simulink model "PubIfDecisionLM_MDL"  (R2020b)
settings: configuration reference "DspaceConfig" (kept outside this file)
PostLoadFcn:
  | if any(exist('dsrtsu_mdlpostloadfcn', 'file') ~= 0), dsrtsu_mdlpostloadfcn('Execute', bdroot); end
InitFcn:
  | , if any(exist('dsmpb_private', 'file') ~= 0), dsmpb_private('dsmpb_mdlclblib', 'Init', bdroot); end,
undefined symbols (not defined in the file or in its folder): OFM_OBJ_FUSIONTYPE_E, OFM_OBJ_MOVINGSTATE_E, OFM_OBJ_ORIENTATION_E, OFM_OBJ_TYPE_E, P_LM_Cyc, P_LM_EMLHistKapRcdBufSize, P_LM_EMLHistTrajBaseDis, P_LM_EMLHistTrajPNum, P_LM_EMLKapCorrMaxThre, P_LM_EMLMinKapThre, P_LM_EMLPathDisDiffThre, P_LM_EMLQuaFiltPar, P_LM_EMLTurnActKapThre, P_LM_EMLValidQuaThre, P_LM_FntPath1Disgap, P_LM_FntPath1MinDis, P_LM_FntPath1Timegap, P_LM_FntPath2Disgap, P_LM_FntPath2MinDis, P_LM_FntPath2Timegap, P_LM_FntPath3Disgap, P_LM_FntPath3MinDis, P_LM_FntPath3Timegap, P_LM_FusBLParFiltP, P_LM_FusEVDifC2Thre, P_LM_FusEVOPath1AllVSLDisThre, P_LM_FusEVOPath1AllVSLLostNumThre, P_LM_FusEVOPath1AllVSLQuaThre, P_LM_FusEVOPath1OTLFacNLC, P_LM_FusOTLQuaThre, P_LM_FusOTLSW, P_LM_FusParC0Index, P_LM_FusParC1Index, P_LM_FusParC2Index, P_LM_FusParC3Index, P_LM_FusVSLQuaThre, P_LM_FusVSLSW, P_LM_FusVSLValidSteerWheerAngThre, P_LM_FusVSLValidVxvThre, P_LM_LaneWidth, P_LM_OTLBufTPInfoEvaFactor, P_LM_OTLObjNum, P_LM_OTLObjSelectAgeThre, P_LM_OTLObjSelectDxAssessVx, P_LM_OTLObjSelectDxThre, P_LM_OTLObjSelectVxThre, P_LM_OTLObjSelectVyAssessDx, P_LM_OTLObjSelectVyThre, P_LM_OTLTrajPntBaseDis, P_LM_OTLTrajStdThre, P_LM_VSLAvailLineNum, P_LM_VSLBLSDiffThre, P_LM_VSLBLSDisRatio, P_LM_VSLFusBLParFiltP_C1, P_LM_VSLFusBLParFiltP_C2, P_LM_VSLFusBLParFiltP_C3, P_LM_VSLFusBLParFiltP_Quality, P_LM_VSLHistTrajBaseDis, P_LM_VSLHistTrajPNum, P_LM_VSLLCC0diff ... (+18)
libraries: simulink x145, LM_LIB x43
(part 9 of 24)

== system PubIfDecisionLM_MDL/Subsystem2/LM_OTL/LM_OTL_MovObjTrajRecord3/LM_OTL_BufRcdObjLostJudge/LM_OTL_RigLaRcdObjLostJudge ==
  Object_ID : Inport  BusOutputAsStruct=on
  LM_OTLRcdObjIDVectK1 : Inport  Port=2
  LM_OTLInterestObjIndexVect : Inport  Port=3
  Bus Selector : BusSelector  OutputSignals=LM_OTLCurRigLaObj1Index,LM_OTLCurRigLaObj2Index
  Bus Selector1 : BusSelector  OutputSignals=LM_OTLBufObjIDInfo.LM_OTLBufR1ObjID,LM_OTLBufObjIDInfo.LM_OTLBufR2ObjID
  Compare To Zero : simulink/Logic and Bit Operations/Compare To Zero  relop===  OutDataTypeStr=boolean
  Compare To Zero1 : simulink/Logic and Bit Operations/Compare To Zero  relop===  OutDataTypeStr=boolean
  Compare To Zero2 : simulink/Logic and Bit Operations/Compare To Zero  relop=~=  OutDataTypeStr=boolean
  Compare To Zero3 : simulink/Logic and Bit Operations/Compare To Zero  relop===  OutDataTypeStr=boolean
  Constant : Constant  OutDataTypeStr=uint8
  Constant1 : Constant  OutDataTypeStr=uint8
  Constant2 : Constant  Value=0  OutDataTypeStr=boolean
  Constant3 : Constant  Value=0  OutDataTypeStr=boolean
  Constant4 : Constant  Value=0  OutDataTypeStr=uint8
  Index Vector2 : MultiPortSwitch  Inputs=1
  Index Vector3 : MultiPortSwitch  Inputs=1
  Logical Operator : Logic  Operator=OR  AllPortsSameDT=off  OutDataTypeStr=boolean
  Logical Operator1 : Logic  Operator=OR  AllPortsSameDT=off  OutDataTypeStr=boolean
  Logical Operator2 : Logic  Operator=NOT  AllPortsSameDT=off  OutDataTypeStr=boolean
  Logical Operator3 : Logic  Operator=NOT  AllPortsSameDT=off  OutDataTypeStr=boolean
  Relational Operator{,1..3} (4 alike) : RelationalOperator  Operator===  OutDataTypeStr=boolean  RndMeth=Simplest
  Switch{,1..5} (6 alike) : Switch  Criteria=u2 ~= 0
  LM_OTLBufRig1ObjLostFlg : Outport
  LM_OTLBufRig2ObjLostFlg : Outport  Port=2
  wires:
  Constant3/1 -> Switch5/1
  Switch5/1 -> LM_OTLBufRig1ObjLostFlg/1  "LM_OTLBufRig1ObjLostFlg"
  Compare To Zero3/1 -> Switch5/2
  Constant2/1 -> Switch4/3
  Compare To Zero2/1 -> Switch4/2
  Switch4/1 -> LM_OTLBufRig2ObjLostFlg/1  "LM_OTLBufRig2ObjLostFlg"
  LM_OTLRcdObjIDVectK1/1 -> Bus Selector1/1
  Constant1/1 -> Switch2/1
  Index Vector3/1 -> Switch3/3
  Compare To Zero1/1 -> Switch2/2, Switch3/2
  Bus Selector/2 -> Compare To Zero1/1, Switch2/3  "<LM_OTLCurRigLaObj2Index>"
  Index Vector2/1 -> Switch1/3
  Constant4/1 -> Switch1/1, Switch3/1
  LM_OTLInterestObjIndexVect/1 -> Bus Selector/1
  Compare To Zero/1 -> Switch1/2, Switch/2
  Switch/1 -> Index Vector2/1
  Switch1/1 -> Relational Operator/1, Relational Operator1/1  "LM_Rig1ObjID"
  Logical Operator3/1 -> Switch5/3
  Object_ID/1 -> Index Vector2/2, Index Vector3/2
  Constant/1 -> Switch/1
  Bus Selector1/1 -> Relational Operator2/2, Relational Operator/2, Compare To Zero3/1  "<LM_OTLBufR1ObjID>"
  Switch3/1 -> Relational Operator2/1, Relational Operator3/1  "LM_Rig2ObjID"
  Bus Selector/1 -> Compare To Zero/1, Switch/3  "<LM_OTLCurRigLaObj1Index>"
  Bus Selector1/2 -> Compare To Zero2/1, Relational Operator3/2, Relational Operator1/2  "<LM_OTLBufR2ObjID>"
  Switch2/1 -> Index Vector3/1
  Relational Operator/1 -> Logical Operator/1
  Logical Operator2/1 -> Switch4/1
  Relational Operator2/1 -> Logical Operator/2
  Relational Operator1/1 -> Logical Operator1/1
  Relational Operator3/1 -> Logical Operator1/2
  Logical Operator1/1 -> Logical Operator2/1
  Logical Operator/1 -> Logical Operator3/1

== system PubIfDecisionLM_MDL/Subsystem2/LM_OTL/LM_OTL_MovObjTrajRecord3/LM_OTL_BufTPCC/Subsystem ==
  VehStandstill : Inport
  LM_OTLOffsetX : Inport  Port=2
  LM_OTLOffsetY : Inport  Port=3
  LM_OTLOffsetAng : Inport  Port=4
  LM_OTLBufL1DxVectK1 : Inport  Port=5
  LM_OTLBufL1DyVectK1 : Inport  Port=6
  LM_OTLBufL2DxVectK1 : Inport  Port=7
  LM_OTLBufL2DyVectK1 : Inport  Port=8
  LM_OTLBufE1DxVectK1 : Inport  Port=9
  LM_OTLBufE1DyVectK1 : Inport  Port=10
  LM_OTLBufE2DxVectK1 : Inport  Port=11
  LM_OTLBufE2DyVectK1 : Inport  Port=12
  LM_OTLBufR1DxVectK1 : Inport  Port=13
  LM_OTLBufR1DyVectK1 : Inport  Port=14
  LM_OTLBufR2DxVectK1 : Inport  Port=15
  LM_OTLBufR2DyVectK1 : Inport  Port=16
  LM_OTLHostBufCoordinateConvert : Subsystem
  LM_OTLLeBufCoordinateConvert : Subsystem
  LM_OTLRiBufCoordinateConvert : Subsystem
  LM_OTLBufL1DxVectK1Adju : Outport
  LM_OTLBufL1DyVectK1Adju : Outport  Port=2
  LM_OTLBufL2DxVectK1Adju : Outport  Port=3
  LM_OTLBufL2DyVectK1Adju : Outport  Port=4
  LM_OTLBufE1DxVectK1Adju : Outport  Port=5
  LM_OTLBufE1DyVectK1Adju : Outport  Port=6
  LM_OTLBufE2DxVectK1Adju : Outport  Port=7
  LM_OTLBufE2DyVectK1Adju : Outport  Port=8
  LM_OTLBufR1DxVectK1Adju : Outport  Port=9
  LM_OTLBufR1DyVectK1Adju : Outport  Port=10
  LM_OTLBufR2DxVectK1Adju : Outport  Port=11
  LM_OTLBufR2DyVectK1Adju : Outport  Port=12
  wires:
  LM_OTLOffsetAng/1 -> LM_OTLLeBufCoordinateConvert/4(LM_OTLOffsetAng), LM_OTLHostBufCoordinateConvert/4(LM_OTLOffsetAng), LM_OTLRiBufCoordinateConvert/4(LM_OTLOffsetAng)
  LM_OTLBufL2DxVectK1/1 -> LM_OTLLeBufCoordinateConvert/7(LM_OTLBufL2DxVectK1)
  LM_OTLOffsetX/1 -> LM_OTLLeBufCoordinateConvert/2(LM_OTLOffsetX), LM_OTLHostBufCoordinateConvert/2(LM_OTLOffsetX), LM_OTLRiBufCoordinateConvert/2(LM_OTLOffsetX)
  LM_OTLBufE2DxVectK1/1 -> LM_OTLHostBufCoordinateConvert/7(LM_OTLBufE2DxVectK1)
  LM_OTLHostBufCoordinateConvert/3(LM_OTLBufE2DxVectK1Adju) -> LM_OTLBufE2DxVectK1Adju/1
  LM_OTLLeBufCoordinateConvert/1(LM_OTLBufL1DxVectK1Adju) -> LM_OTLBufL1DxVectK1Adju/1
  VehStandstill/1 -> LM_OTLRiBufCoordinateConvert/1(VehStandstill), LM_OTLHostBufCoordinateConvert/1(VehStandstill), LM_OTLLeBufCoordinateConvert/1(VehStandstill)
  LM_OTLBufR2DyVectK1/1 -> LM_OTLRiBufCoordinateConvert/8(LM_OTLBufR2DyVectK1)
  LM_OTLLeBufCoordinateConvert/4(LM_OTLBufL2DyVectK1Adju) -> LM_OTLBufL2DyVectK1Adju/1
  LM_OTLBufE1DxVectK1/1 -> LM_OTLHostBufCoordinateConvert/5(LM_OTLBufE1DxVectK1)
  LM_OTLBufR2DxVectK1/1 -> LM_OTLRiBufCoordinateConvert/7(LM_OTLBufR2DxVectK1)
  LM_OTLBufE1DyVectK1/1 -> LM_OTLHostBufCoordinateConvert/6(LM_OTLBufE1DyVectK1)
  LM_OTLRiBufCoordinateConvert/3(LM_OTLBufR2DxVectK1Adju) -> LM_OTLBufR2DxVectK1Adju/1
  LM_OTLHostBufCoordinateConvert/4(LM_OTLBufE2DyVectK1Adju) -> LM_OTLBufE2DyVectK1Adju/1
  LM_OTLRiBufCoordinateConvert/4(LM_OTLBufR2DyVectK1Adju) -> LM_OTLBufR2DyVectK1Adju/1
  LM_OTLBufL1DyVectK1/1 -> LM_OTLLeBufCoordinateConvert/6(LM_OTLBufL1DyVectK1)
  LM_OTLBufR1DxVectK1/1 -> LM_OTLRiBufCoordinateConvert/5(LM_OTLBufR1DxVectK1)
  LM_OTLOffsetY/1 -> LM_OTLHostBufCoordinateConvert/3(LM_OTLOffsetY), LM_OTLRiBufCoordinateConvert/3(LM_OTLOffsetY), LM_OTLLeBufCoordinateConvert/3(LM_OTLOffsetY)
  LM_OTLBufR1DyVectK1/1 -> LM_OTLRiBufCoordinateConvert/6(LM_OTLBufR1DyVectK1)
  LM_OTLBufL2DyVectK1/1 -> LM_OTLLeBufCoordinateConvert/8(LM_OTLBufL2DyVectK1)
  LM_OTLHostBufCoordinateConvert/1(LM_OTLBufE1DxVectK1Adju) -> LM_OTLBufE1DxVectK1Adju/1
  LM_OTLRiBufCoordinateConvert/1(LM_OTLBufR1DxVectK1Adju) -> LM_OTLBufR1DxVectK1Adju/1
  LM_OTLLeBufCoordinateConvert/3(LM_OTLBufL2DxVectK1Adju) -> LM_OTLBufL2DxVectK1Adju/1
  LM_OTLRiBufCoordinateConvert/2(LM_OTLBufR1DyVectK1Adju) -> LM_OTLBufR1DyVectK1Adju/1
  LM_OTLHostBufCoordinateConvert/2(LM_OTLBufE1DyVectK1Adju) -> LM_OTLBufE1DyVectK1Adju/1
  LM_OTLLeBufCoordinateConvert/2(LM_OTLBufL1DyVectK1Adju) -> LM_OTLBufL1DyVectK1Adju/1
  LM_OTLBufE2DyVectK1/1 -> LM_OTLHostBufCoordinateConvert/8(LM_OTLBufE2DyVectK1)
  LM_OTLBufL1DxVectK1/1 -> LM_OTLLeBufCoordinateConvert/5(LM_OTLBufL1DxVectK1)

== system PubIfDecisionLM_MDL/Subsystem2/LM_OTL/LM_OTL_MovObjTrajRecord3/LM_OTL_MovObjSelc/LM_OTL_MovObjInterestedSelc ==
  LM_OTL_MovObjValid : Inport
  P_LM_ObjNum : Inport  Port=2
  Object_DX : Inport  Port=3
  Object_DY : Inport  Port=4
  For Iterator : ForIterator  IterationSource=external
  LM_OTL_ObjSelcIndexCalc : Subsystem
  LM_OTL_ObjSelcIndexCheck : Subsystem
  LM_OTL_ObjSelcInfoCalc : Subsystem
  LM_OTLLeObj1Index : Outport
  LM_OTLLeObj2Index : Outport  Port=2
  LM_OTLHostObj1Index : Outport  Port=3
  LM_OTLHostObj2Index : Outport  Port=4
  LM_OTLRigObj1Index : Outport  Port=5
  LM_OTLRigObj2Index : Outport  Port=6
  wires:
  LM_OTL_ObjSelcIndexCheck/3(LM_OTLHostObj1Index) -> LM_OTLHostObj1Index/1
  [ObjDy] -> LM_OTL_ObjSelcIndexCheck/8(Object_DX)
  [ObjValid] -> LM_OTL_ObjSelcIndexCheck/7(LM_OTL_MovObjValid)
  LM_OTL_ObjSelcIndexCalc/6(RigObj2CheckInfo) -> LM_OTL_ObjSelcIndexCheck/6(RigObj2CheckInfo)
  LM_OTL_ObjSelcIndexCalc/5(RigObj1CheckInfo) -> LM_OTL_ObjSelcIndexCheck/5(RigObj1CheckInfo)
  LM_OTL_ObjSelcIndexCalc/4(HostObj2CheckInfo) -> LM_OTL_ObjSelcIndexCheck/4(HostObj2CheckInfo)
  LM_OTL_ObjSelcIndexCalc/3(HostObj1CheckInfo) -> LM_OTL_ObjSelcIndexCheck/3(HostObj1CheckInfo)
  LM_OTL_ObjSelcIndexCalc/2(LeObj2CheckInfo) -> LM_OTL_ObjSelcIndexCheck/2(LeObj2CheckInfo)
  LM_OTL_ObjSelcIndexCalc/1(LeObj1CheckInfo) -> LM_OTL_ObjSelcIndexCheck/1(LeObj1CheckInfo)
  LM_OTL_ObjSelcIndexCheck/6(LM_OTLRigObj2Index) -> LM_OTLRigObj2Index/1
  LM_OTL_ObjSelcIndexCheck/5(LM_OTLRigObj1Index) -> LM_OTLRigObj1Index/1
  LM_OTL_ObjSelcIndexCheck/4(LM_OTLHostObj2Index) -> LM_OTLHostObj2Index/1
  LM_OTL_ObjSelcIndexCheck/2(LM_OTLLeObj2Index) -> LM_OTLLeObj2Index/1
  LM_OTL_ObjSelcIndexCheck/1(LM_OTLLeObj1Index) -> LM_OTLLeObj1Index/1
  LM_OTL_ObjSelcInfoCalc/2(ObjSelcDyInfo) -> LM_OTL_ObjSelcIndexCalc/2(ObjSelcDyInfo)
  LM_OTL_ObjSelcInfoCalc/1(ObjSelcDxInfo) -> LM_OTL_ObjSelcIndexCalc/1(ObjSelcDxInfo)
  Object_DY/1 -> LM_OTL_ObjSelcInfoCalc/3(Object_DY), [ObjDy]
  Object_DX/1 -> LM_OTL_ObjSelcInfoCalc/2(Object_DX)
  LM_OTL_MovObjValid/1 -> LM_OTL_ObjSelcInfoCalc/1(ILM_OTL_MovObjValid), [ObjValid]
  For Iterator/1 -> LM_OTL_ObjSelcInfoCalc/4(C_LM_ObjNum), LM_OTL_ObjSelcIndexCalc/3(C_LM_ObjNum)
  P_LM_ObjNum/1 -> For Iterator/1

== system PubIfDecisionLM_MDL/Subsystem2/LM_OTL/LM_OTL_MovObjTrajRecord3/LM_OTL_MovObjSelc/Subsystem3 ==
  vxvRefMs : Inport
  <Object_ID> : Inport  Port=2  Partition=on  PartitionDimension=1  PartitionWidth=1  PartitionOffset=0
  <Object_Type> : Inport  Port=3  Partition=on  PartitionDimension=1  PartitionWidth=1  PartitionOffset=0
  <Object_MovingState> : Inport  Port=4  Partition=on  PartitionDimension=1  PartitionWidth=1  PartitionOffset=0
  <Object_VX> : Inport  Port=5  Partition=on  PartitionDimension=1  PartitionWidth=1  PartitionOffset=0
  <Object_Orientation> : Inport  Port=6  Partition=on  PartitionDimension=1  PartitionWidth=1  PartitionOffset=0
  <Object_Fus_Type> : Inport  Port=7  Partition=on  PartitionDimension=1  PartitionWidth=1  PartitionOffset=0
  <Object_ExistProb> : Inport  Port=8  Partition=on  PartitionDimension=1  PartitionWidth=1  PartitionOffset=0
  <Object_VY> : Inport  Port=9  Partition=on  PartitionDimension=1  PartitionWidth=1  PartitionOffset=0
  <Object_DX> : Inport  Port=10  Partition=on  PartitionDimension=1  PartitionWidth=1  PartitionOffset=0
  <Object_Age> : Inport  Port=11  Partition=on  PartitionDimension=1  PartitionWidth=1  PartitionOffset=0
  For Each : ForEach  DisableCoverage=on
  ILM_OTL_MovObjSelectDeFault : Subsystem  TreatAsAtomicUnit=on
  If : If  IfExpression=u1
  LM_OTL_MovObjSelect : Subsystem  TreatAsAtomicUnit=on
  Merge : Merge
  ObjIsInvalidCalc : Subsystem
  LM_OTL_MovObjValid : Outport  ConcatenationDimension=1
  wires:
  <Object_Type>/1 -> LM_OTL_MovObjSelect/2(Object_Type)
  <Object_VY>/1 -> LM_OTL_MovObjSelect/8(Object_VY)
  <Object_VX>/1 -> LM_OTL_MovObjSelect/4(Object_VX)
  <Object_DX>/1 -> LM_OTL_MovObjSelect/9(Object_DX)
  <Object_ID>/1 -> ObjIsInvalidCalc/1(ObjectID)
  <Object_MovingState>/1 -> LM_OTL_MovObjSelect/3(Object_MovingState)
  <Object_Fus_Type>/1 -> LM_OTL_MovObjSelect/6(Object_Fus_Type)
  ILM_OTL_MovObjSelectDeFault/1(LM_OTL_MovObjValid) -> Merge/1
  If/1 -> ILM_OTL_MovObjSelectDeFault/Action
  <Object_Age>/1 -> LM_OTL_MovObjSelect/10(Object_Age)
  If/2 -> LM_OTL_MovObjSelect/Action
  LM_OTL_MovObjSelect/1(LM_OTL_MovObjValid) -> Merge/2
  ObjIsInvalidCalc/1(ObjIsInvalid) -> If/1
  <Object_Orientation>/1 -> LM_OTL_MovObjSelect/5(Object_Orientation)
  <Object_ExistProb>/1 -> LM_OTL_MovObjSelect/7(Object_ExistProb)
  Merge/1 -> LM_OTL_MovObjValid/1
  vxvRefMs/1 -> LM_OTL_MovObjSelect/1(vxvRefMs)

== system PubIfDecisionLM_MDL/Subsystem2/LM_OTL/LM_OTL_MovObjTrajRecord3/LM_OTL_ObjAlreadyRcdedJudge/LM_OTL_CurObjIDCalc ==
  Object_ID : Inport  BusOutputAsStruct=on
  LM_OTLCurLeLaObj1Index : Inport  Port=2
  LM_OTLCurLeLaObj2Index : Inport  Port=3
  LM_OTLCurEgoLaObj1Index : Inport  Port=4
  LM_OTLCurEgoLaObj2Index : Inport  Port=5
  LM_OTLCurRigLaObj1Index : Inport  Port=6
  LM_OTLCurRigLaObj2Index : Inport  Port=7
  LM_OTL_CurEgoLaObjID : Subsystem
  LM_OTL_CurLeLaObjID : Subsystem
  LM_OTL_RigEgoLaObjID : Subsystem
  LM_OTLCurLeLaObj1ID : Outport
  LM_OTLCurLeLaObj2ID : Outport  Port=2
  LM_OTLCurEgoLaObj1ID : Outport  Port=3
  LM_OTLCurEgoLaObj2ID : Outport  Port=4
  LM_OTLCurRigLaObj1ID : Outport  Port=5
  LM_OTLCurRigLaObj2ID : Outport  Port=6
  wires:
  LM_OTL_CurLeLaObjID/2(LM_OTLCurLeLaObj2ID) -> LM_OTLCurLeLaObj2ID/1
  LM_OTL_CurEgoLaObjID/2(LM_OTLCurEgoLaObj2ID) -> LM_OTLCurEgoLaObj2ID/1
  LM_OTL_CurEgoLaObjID/1(LM_OTLCurEgoLaObj1ID) -> LM_OTLCurEgoLaObj1ID/1
  LM_OTL_RigEgoLaObjID/1(LM_OTLCurRigLaObj1ID) -> LM_OTLCurRigLaObj1ID/1
  LM_OTL_RigEgoLaObjID/2(LM_OTLCurRigLaObj2ID) -> LM_OTLCurRigLaObj2ID/1
  LM_OTL_CurLeLaObjID/1(LM_OTLCurLeLaObj1ID) -> LM_OTLCurLeLaObj1ID/1
  Object_ID/1 -> LM_OTL_RigEgoLaObjID/1(Object_ID), LM_OTL_CurEgoLaObjID/1(Object_ID), LM_OTL_CurLeLaObjID/1(Object_ID)
  LM_OTLCurLeLaObj2Index/1 -> LM_OTL_CurLeLaObjID/3(LM_OTLCurLeLaObj2Index)
  LM_OTLCurLeLaObj1Index/1 -> LM_OTL_CurLeLaObjID/2(LM_OTLCurLeLaObj1Index)
  LM_OTLCurEgoLaObj1Index/1 -> LM_OTL_CurEgoLaObjID/2(LM_OTLCurEgoLaObj1Index)
  LM_OTLCurEgoLaObj2Index/1 -> LM_OTL_CurEgoLaObjID/3(LM_OTLCurEgoLaObj2Index)
  LM_OTLCurRigLaObj1Index/1 -> LM_OTL_RigEgoLaObjID/2(LM_OTLCurRigLaObj1Index)
  LM_OTLCurRigLaObj2Index/1 -> LM_OTL_RigEgoLaObjID/3(LM_OTLCurRigLaObj2Index)

== system PubIfDecisionLM_MDL/Subsystem2/LM_OTL/LM_OTL_MovObjTrajRecord3/LM_OTL_ObjAlreadyRcdedJudge/LM_OTL_EglLaneRcdJudge ==
  LM_OTLCurEgoLa1ObjID : Inport
  LM_OTLCurEgoLa2ObjID : Inport  Port=2
  LM_OTLBufE1ObjIDK1 : Inport  Port=3
  LM_OTLBufE2ObjIDK1 : Inport  Port=4
  Compare To Zero : simulink/Logic and Bit Operations/Compare To Zero  relop===  OutDataTypeStr=boolean
  Compare To Zero1 : simulink/Logic and Bit Operations/Compare To Zero  relop===  OutDataTypeStr=boolean
  Constant{1..2,6,9} (4 alike) : Constant  Value=0  OutDataTypeStr=uint8
  Constant4 : Constant  OutDataTypeStr=uint8
  Constant5 : Constant  Value=2  OutDataTypeStr=uint8
  Constant7 : Constant  OutDataTypeStr=uint8
  Constant8 : Constant  Value=2  OutDataTypeStr=uint8
  Relational Operator{,1..3} (4 alike) : RelationalOperator  Operator===  OutDataTypeStr=boolean  RndMeth=Simplest
  Switch{,1..5} (6 alike) : Switch  Criteria=u2 ~= 0
  LM_OTLCurEgoLaObj1RcdedFlg : Outport
  LM_OTLCurEgoLaObj2RcdedFlg : Outport  Port=2
  wires:
  Switch2/1 -> Switch5/3  "LM_OTLCurEgoLaObj2RcdedFlg"
  Constant2/1 -> Switch5/1
  Compare To Zero1/1 -> Switch5/2
  Switch/1 -> Switch4/3  "LM_OTLCurEgoLaObj1RcdedFlg"
  LM_OTLCurEgoLa1ObjID/1 -> Relational Operator/1, Relational Operator1/1, Compare To Zero/1  "LM_Le1ObjID"
  Compare To Zero/1 -> Switch4/2
  Constant1/1 -> Switch4/1
  Switch5/1 -> LM_OTLCurEgoLaObj2RcdedFlg/1  "LM_OTLCurEgoLaObj2RcdedFlg"
  LM_OTLBufE2ObjIDK1/1 -> Relational Operator1/2, Relational Operator3/2
  LM_OTLCurEgoLa2ObjID/1 -> Compare To Zero1/1, Relational Operator3/1, Relational Operator2/1  "HostLa2ObjID"
  LM_OTLBufE1ObjIDK1/1 -> Relational Operator2/2, Relational Operator/2
  Switch4/1 -> LM_OTLCurEgoLaObj1RcdedFlg/1  "LM_OTLCurEgoLaObj1RcdedFlg"
  Constant5/1 -> Switch1/1
  Relational Operator1/1 -> Switch1/2
  Constant4/1 -> Switch/1
  Relational Operator2/1 -> Switch2/2
  Relational Operator3/1 -> Switch3/2
  Switch1/1 -> Switch/3
  Constant6/1 -> Switch1/3
  Constant7/1 -> Switch2/1
  Constant9/1 -> Switch3/3
  Constant8/1 -> Switch3/1
  Relational Operator/1 -> Switch/2
  Switch3/1 -> Switch2/3

== system PubIfDecisionLM_MDL/Subsystem2/LM_OTL/LM_OTL_MovObjTrajRecord3/LM_OTL_ObjAlreadyRcdedJudge/LM_OTL_LeLaneRcdJudge ==
  LM_OTLCurLeLa1ObjID : Inport
  LM_OTLCurLeLa2ObjID : Inport  Port=2
  LM_OTLBufL1ObjIDK1 : Inport  Port=3
  LM_OTLBufL2ObjIDK1 : Inport  Port=4
  Compare To Zero : simulink/Logic and Bit Operations/Compare To Zero  relop===  OutDataTypeStr=boolean
  Compare To Zero1 : simulink/Logic and Bit Operations/Compare To Zero  relop===  OutDataTypeStr=boolean
  Constant{1..2,6,9} (4 alike) : Constant  Value=0  OutDataTypeStr=uint8
  Constant4 : Constant  OutDataTypeStr=uint8
  Constant5 : Constant  Value=2  OutDataTypeStr=uint8
  Constant7 : Constant  OutDataTypeStr=uint8
  Constant8 : Constant  Value=2  OutDataTypeStr=uint8
  Relational Operator{,1..3} (4 alike) : RelationalOperator  Operator===  OutDataTypeStr=boolean  RndMeth=Simplest
  Switch{,1..5} (6 alike) : Switch  Criteria=u2 ~= 0
  LM_OTLCurLeLaObj1RcdedFlg : Outport
  LM_OTLCurLeLaObj2RcdedFlg : Outport  Port=2
  wires:
  Switch2/1 -> Switch5/3  "LM_OTLCurLeLaObj2RcdedFlg"
  Constant2/1 -> Switch5/1
  Compare To Zero1/1 -> Switch5/2
  Switch/1 -> Switch4/3  "LM_OTLCurLeLaObj1RcdedFlg"
  Constant1/1 -> Switch4/1
  Compare To Zero/1 -> Switch4/2
  LM_OTLCurLeLa1ObjID/1 -> Relational Operator1/1, Relational Operator/1, Compare To Zero/1  "LM_Le1ObjID"
  Switch4/1 -> LM_OTLCurLeLaObj1RcdedFlg/1  "LM_OTLCurLeLaObj1RcdedFlg"
  LM_OTLBufL1ObjIDK1/1 -> Relational Operator/2, Relational Operator2/2
  LM_OTLCurLeLa2ObjID/1 -> Relational Operator3/1, Compare To Zero1/1, Relational Operator2/1  "LM_Le2ObjID"
  LM_OTLBufL2ObjIDK1/1 -> Relational Operator3/2, Relational Operator1/2
  Relational Operator/1 -> Switch/2
  Switch5/1 -> LM_OTLCurLeLaObj2RcdedFlg/1  "LM_OTLCurLeLaObj2RcdedFlg"
  Constant4/1 -> Switch/1
  Relational Operator1/1 -> Switch1/2
  Constant5/1 -> Switch1/1
  Constant6/1 -> Switch1/3
  Switch1/1 -> Switch/3
  Switch3/1 -> Switch2/3
  Constant9/1 -> Switch3/3
  Constant8/1 -> Switch3/1
  Relational Operator3/1 -> Switch3/2
  Constant7/1 -> Switch2/1
  Relational Operator2/1 -> Switch2/2

== system PubIfDecisionLM_MDL/Subsystem2/LM_OTL/LM_OTL_MovObjTrajRecord3/LM_OTL_ObjAlreadyRcdedJudge/LM_OTL_RigLaneRcdJudge ==
  LM_OTLCurRigLa1ObjID : Inport
  LM_OTLCurRigLa2ObjID : Inport  Port=2
  LM_OTLBufR1ObjIDK1 : Inport  Port=3
  LM_OTLBufR2ObjIDK1 : Inport  Port=4
  Compare To Zero : simulink/Logic and Bit Operations/Compare To Zero  relop===  OutDataTypeStr=boolean
  Compare To Zero1 : simulink/Logic and Bit Operations/Compare To Zero  relop===  OutDataTypeStr=boolean
  Constant{1..2,6,9} (4 alike) : Constant  Value=0  OutDataTypeStr=uint8
  Constant4 : Constant  OutDataTypeStr=uint8
  Constant5 : Constant  Value=2  OutDataTypeStr=uint8
  Constant7 : Constant  OutDataTypeStr=uint8
  Constant8 : Constant  Value=2  OutDataTypeStr=uint8
  Relational Operator{,1..3} (4 alike) : RelationalOperator  Operator===  OutDataTypeStr=boolean  RndMeth=Simplest
  Switch{,1..5} (6 alike) : Switch  Criteria=u2 ~= 0
  LM_OTLCurRigLaObj1RcdedFlg : Outport
  LM_OTLCurRigLaObj2RcdedFlg : Outport  Port=2
  wires:
  Switch2/1 -> Switch5/3  "LM_OTLCurRigLaObj2RcdedFlg"
  Constant2/1 -> Switch5/1
  Compare To Zero1/1 -> Switch5/2
  Switch/1 -> Switch4/3  "LM_OTLCurRigLaObj1RcdedFlg"
  LM_OTLCurRigLa1ObjID/1 -> Relational Operator1/1, Relational Operator/1, Compare To Zero/1
  Compare To Zero/1 -> Switch4/2
  Constant1/1 -> Switch4/1
  Switch4/1 -> LM_OTLCurRigLaObj1RcdedFlg/1  "LM_OTLCurRigLaObj1RcdedFlg"
  LM_OTLBufR1ObjIDK1/1 -> Relational Operator2/2, Relational Operator/2
  LM_OTLCurRigLa2ObjID/1 -> Relational Operator3/1, Relational Operator2/1, Compare To Zero1/1  "Rig2ObjID"
  LM_OTLBufR2ObjIDK1/1 -> Relational Operator3/2, Relational Operator1/2
  Switch5/1 -> LM_OTLCurRigLaObj2RcdedFlg/1  "LM_OTLCurRigLaObj2RcdedFlg"
  Constant5/1 -> Switch1/1
  Relational Operator1/1 -> Switch1/2
  Constant4/1 -> Switch/1
  Relational Operator2/1 -> Switch2/2
  Relational Operator3/1 -> Switch3/2
  Switch1/1 -> Switch/3
  Constant6/1 -> Switch1/3
  Constant7/1 -> Switch2/1
  Constant9/1 -> Switch3/3
  Constant8/1 -> Switch3/1
  Relational Operator/1 -> Switch/2
  Switch3/1 -> Switch2/3

== system PubIfDecisionLM_MDL/Subsystem2/LM_OTL/LM_OTL_MovObjTrajRecord3/LM_OTL_ObjRcdFlgJudge/LM_OTL_BufObjEndDxCalc ==
  LM_OTLBufLe1ObjDxVectK1 : Inport
  LM_OTLBufLe2ObjDxVectK1 : Inport  Port=2
  LM_OTLBufEgo1ObjDxVectK1 : Inport  Port=3
  LM_OTLBufEgo2ObjDxVectK1 : Inport  Port=4
  LM_OTLBufRig1ObjDxVectK1 : Inport  Port=5
  LM_OTLBufRig2ObjDxVectK1 : Inport  Port=6
  LM_OTLBufLe1ObjPEndIndexK1 : Inport  Port=7
  LM_OTLBufLe2ObjPEndIndexK1 : Inport  Port=8
  LM_OTLBufEgo1ObjPEndIndexK1 : Inport  Port=9
  LM_OTLBufEgo2ObjPEndIndexK1 : Inport  Port=10
  LM_OTLBufRig1ObjPEndIndexK1 : Inport  Port=11
  LM_OTLBufRig2ObjPEndIndexK1 : Inport  Port=12
  Compare To Zero{,1..5} (6 alike) : simulink/Logic and Bit Operations/Compare To Zero  relop===  OutDataTypeStr=boolean
  Constant{,1..5} (6 alike) : Constant  OutDataTypeStr=uint8
  Index Vector{,1..5} (6 alike) : MultiPortSwitch  Inputs=1
  Switch{,1..5} (6 alike) : Switch  Criteria=u2 ~= 0
  LM_OTLBufLe1ObjDxK1 : Outport
  LM_OTLBufLe2ObjDxK1 : Outport  Port=2
  LM_OTLBufEgo1ObjDxK1 : Outport  Port=3
  LM_OTLBufEgo2ObjDxK1 : Outport  Port=4
  LM_OTLBufRig1ObjDxK1 : Outport  Port=5
  LM_OTLBufRig2ObjDxK1 : Outport  Port=6
  wires:
  LM_OTLBufLe1ObjDxVectK1/1 -> Index Vector/2
  LM_OTLBufLe1ObjPEndIndexK1/1 -> Switch/3, Compare To Zero/1
  LM_OTLBufLe2ObjDxVectK1/1 -> Index Vector1/2
  Compare To Zero/1 -> Switch/2
  Constant/1 -> Switch/1
  Switch/1 -> Index Vector/1
  Switch1/1 -> Index Vector1/1
  Constant1/1 -> Switch1/1
  Compare To Zero1/1 -> Switch1/2
  LM_OTLBufLe2ObjPEndIndexK1/1 -> Switch1/3, Compare To Zero1/1
  LM_OTLBufEgo2ObjPEndIndexK1/1 -> Compare To Zero3/1, Switch3/3
  Compare To Zero3/1 -> Switch3/2
  Constant3/1 -> Switch3/1
  Switch3/1 -> Index Vector3/1
  Switch2/1 -> Index Vector2/1
  Constant2/1 -> Switch2/1
  Compare To Zero2/1 -> Switch2/2
  LM_OTLBufEgo2ObjDxVectK1/1 -> Index Vector3/2
  LM_OTLBufEgo1ObjPEndIndexK1/1 -> Compare To Zero2/1, Switch2/3
  LM_OTLBufEgo1ObjDxVectK1/1 -> Index Vector2/2
  Index Vector/1 -> LM_OTLBufLe1ObjDxK1/1  "LM_OTLBufLe1ObjDxK1"
  Index Vector1/1 -> LM_OTLBufLe2ObjDxK1/1  "LM_OTLBufLe2ObjDxK1"
  Index Vector3/1 -> LM_OTLBufEgo2ObjDxK1/1  "LM_OTLBufEgo2ObjDxK1"
  Index Vector2/1 -> LM_OTLBufEgo1ObjDxK1/1  "LM_OTLBufEgo1ObjDxK1"
  Index Vector4/1 -> LM_OTLBufRig1ObjDxK1/1  "LM_OTLBufRig1ObjDxK1"
  Index Vector5/1 -> LM_OTLBufRig2ObjDxK1/1  "LM_OTLBufRig2ObjDxK1"
  LM_OTLBufRig1ObjDxVectK1/1 -> Index Vector4/2
  LM_OTLBufRig1ObjPEndIndexK1/1 -> Switch4/3, Compare To Zero4/1
  LM_OTLBufRig2ObjDxVectK1/1 -> Index Vector5/2
  Compare To Zero4/1 -> Switch4/2
  Constant4/1 -> Switch4/1
  Switch4/1 -> Index Vector4/1
  Switch5/1 -> Index Vector5/1
  Constant5/1 -> Switch5/1
  Compare To Zero5/1 -> Switch5/2
  LM_OTLBufRig2ObjPEndIndexK1/1 -> Switch5/3, Compare To Zero5/1

== system PubIfDecisionLM_MDL/Subsystem2/LM_OTL/LM_OTL_MovObjTrajRecord3/LM_OTL_ObjRcdFlgJudge/LM_OTL_CurObjDxCalc ==
  Object_Dx : Inport
  Object_Dy : Inport  Port=2
  LM_OTLCurLeLaObj1Index : Inport  Port=3
  LM_OTLCurLeLaObj2Index : Inport  Port=4
  LM_OTLCurEgoLaObj1Index : Inport  Port=5
  LM_OTLCurEgoLaObj2Index : Inport  Port=6
  LM_OTLCurRigLaObj1Index : Inport  Port=7
  LM_OTLCurRigLaObj2Index : Inport  Port=8
  LM_OTLCurEgoLaObjDxCalc : Subsystem
  LM_OTLCurLeLaObjDxCalc : Subsystem
  LM_OTLCurRigLaObjDxCalc : Subsystem
  LM_OTLCurLeLaObj1Dx : Outport
  LM_OTLCurLeLaObj1Dy : Outport  Port=2
  LM_OTLCurLeLaObj2Dx : Outport  Port=3
  LM_OTLCurLeLaObj2Dy : Outport  Port=4
  LM_OTLCurEgoLaObj1Dx : Outport  Port=5
  LM_OTLCurEgoLaObj1Dy : Outport  Port=6
  LM_OTLCurEgoLaObj2Dx : Outport  Port=7
  LM_OTLCurEgoLaObj2Dy : Outport  Port=8
  LM_OTLCurRigLaObj1Dx : Outport  Port=9
  LM_OTLCurRigLaObj1Dy : Outport  Port=10
  LM_OTLCurRigLaObj2Dx : Outport  Port=11
  LM_OTLCurRigLaObj2Dy : Outport  Port=12
  wires:
  LM_OTLCurRigLaObj2Index/1 -> LM_OTLCurRigLaObjDxCalc/4(LM_OTLCurRigLaObj2Index)
  LM_OTLCurLeLaObj2Index/1 -> LM_OTLCurLeLaObjDxCalc/4(LM_OTLCurLeLaObj2Index)
  Object_Dx/1 -> LM_OTLCurRigLaObjDxCalc/2(Object_Dx), LM_OTLCurEgoLaObjDxCalc/2(Object_Dx), LM_OTLCurLeLaObjDxCalc/2(Object_Dx)
  LM_OTLCurEgoLaObj2Index/1 -> LM_OTLCurEgoLaObjDxCalc/4(LM_OTLCurEgoLaObj2Index)
  LM_OTLCurEgoLaObj1Index/1 -> LM_OTLCurEgoLaObjDxCalc/1(LM_OTLCurEgoLaObj1Index)
  LM_OTLCurRigLaObj1Index/1 -> LM_OTLCurRigLaObjDxCalc/1(LM_OTLCurRigLaObj1Index)
  LM_OTLCurLeLaObjDxCalc/3(LM_OTLCurLeLaObj2Dx) -> LM_OTLCurLeLaObj2Dx/1
  LM_OTLCurLeLaObj1Index/1 -> LM_OTLCurLeLaObjDxCalc/1(LM_OTLCurLeLaObj1Index)
  LM_OTLCurLeLaObjDxCalc/1(LM_OTLCurLeLaObj1Dx) -> LM_OTLCurLeLaObj1Dx/1
  Object_Dy/1 -> LM_OTLCurRigLaObjDxCalc/3(Object_Dy), LM_OTLCurEgoLaObjDxCalc/3(Object_Dy), LM_OTLCurLeLaObjDxCalc/3(Object_Dy)
  LM_OTLCurLeLaObjDxCalc/4(LM_OTLCurLeLaObj2Dy) -> LM_OTLCurLeLaObj2Dy/1
  LM_OTLCurLeLaObjDxCalc/2(LM_OTLCurLeLaObj1Dy) -> LM_OTLCurLeLaObj1Dy/1
  LM_OTLCurEgoLaObjDxCalc/1(LM_OTLCurEgoLaObj1Dx) -> LM_OTLCurEgoLaObj1Dx/1
  LM_OTLCurEgoLaObjDxCalc/2(LM_OTLCurEgoLaObj1Dy) -> LM_OTLCurEgoLaObj1Dy/1
  LM_OTLCurEgoLaObjDxCalc/3(LM_OTLCurEgoLaObj2Dx) -> LM_OTLCurEgoLaObj2Dx/1
  LM_OTLCurEgoLaObjDxCalc/4(LM_OTLCurEgoLaObj2Dy) -> LM_OTLCurEgoLaObj2Dy/1
  LM_OTLCurRigLaObjDxCalc/1(LM_OTLCurRigLaObj1Dx) -> LM_OTLCurRigLaObj1Dx/1
  LM_OTLCurRigLaObjDxCalc/2(LM_OTLCurRigLaObj1Dy) -> LM_OTLCurRigLaObj1Dy/1
  LM_OTLCurRigLaObjDxCalc/3(LM_OTLCurRigLaObj2Dx) -> LM_OTLCurRigLaObj2Dx/1
  LM_OTLCurRigLaObjDxCalc/4(LM_OTLCurRigLaObj2Dy) -> LM_OTLCurRigLaObj2Dy/1

== system PubIfDecisionLM_MDL/Subsystem2/LM_OTL/LM_OTL_MovObjTrajRecord3/LM_OTL_ObjRcdFlgJudge/LM_OTL_EgoLaObjRcdFlgJudge ==
  note: P_LM_OTLTrajPntBaseDis
  LM_OTLCurEgoLaObj1RcdedFlg : Inport
  LM_OTLCurEgoLaObj2RcdedFlg : Inport  Port=2
  LM_OTLCurEgoLaObj1Index : Inport  Port=3
  LM_OTLCurEgoLaObj2Index : Inport  Port=4
  LM_OTLCurEgoLaObj1Dx : Inport  Port=5
  LM_OTLCurEgoLaObj2Dx : Inport  Port=6
  LM_OTLBufEgo1ObjDxK1 : Inport  Port=7
  LM_OTLBufEgo2ObjDxK1 : Inport  Port=8
  Compare To Zero : simulink/Logic and Bit Operations/Compare To Zero  relop===  OutDataTypeStr=boolean
  Compare To Zero1 : simulink/Logic and Bit Operations/Compare To Zero  relop===  OutDataTypeStr=boolean
  Constant : Constant  OutDataTypeStr=uint8
  Constant1 : Constant  Value=P_LM_OTLTrajPntBaseDis
  Constant2 : Constant  Value=2  OutDataTypeStr=uint8
  Constant3 : Constant  OutDataTypeStr=boolean
  Constant4 : Constant  OutDataTypeStr=boolean
  Constant5 : Constant  OutDataTypeStr=uint8
  Constant6 : Constant  Value=2  OutDataTypeStr=uint8
  Constant7 : Constant  Value=0  OutDataTypeStr=boolean
  DocBlock : simulink/Model-Wide Utilities/DocBlock  DocumentType=Text
      content=|
      | 1.功能描述
      |
      |    该模块的主要功能是判断感兴趣目标当前周期是否满足存储条件
      |
      | 2.算法说明
      |
      |    1）当目标索引不为0
      |    1.1）当目标已经在buffer中存储，需要判断当前dx与上一记录dx的差值是否大于等于2m，满足则置存储标志位为1，否则置0
      |    1.2）当目标未在buffer中存储，则直接置存储标志位为1
      |    2）当目标索引为0（即对应车道不存在感兴趣目标）
      |    直接置存储标志位为0
  Relational Operator{,3..5} (4 alike) : RelationalOperator  Operator===  OutDataTypeStr=boolean  RndMeth=Simplest
  Relational Operator{1..2,6..7} (4 alike) : RelationalOperator  OutDataTypeStr=boolean  RndMeth=Simplest
  Subtract{,1..3} (4 alike) : Sum  Inputs=+-
  Switch{,1..4,7} (6 alike) : Switch  Criteria=u2 ~= 0
  LM_OTLCurEgoLaObj1RcdFlg : Outport
  LM_OTLCurEgoLaObj2RcdFlg : Outport  Port=2
  wires:
  Switch2/1 -> Switch7/3  "LM_OTLEgo2ObjRcdValid"
  Compare To Zero1/1 -> Switch7/2
  Switch/1 -> Switch4/3  "LM_OTLEgo1ObjRcdValid"
  Constant7/1 -> Switch4/1, Switch7/1
  Compare To Zero/1 -> Switch4/2
  Subtract3/1 -> Relational Operator7/1
  Subtract2/1 -> Relational Operator6/1
  LM_OTLCurEgoLaObj2Dx/1 -> Subtract2/1, Subtract3/1
  LM_OTLCurEgoLaObj2Index/1 -> Compare To Zero1/1
  LM_OTLCurEgoLaObj2RcdedFlg/1 -> Relational Operator5/1, Relational Operator4/1
  Constant5/1 -> Relational Operator4/2
  Constant6/1 -> Relational Operator5/2
  Switch7/1 -> LM_OTLCurEgoLaObj2RcdFlg/1  "LM_OTLCurEgoLaObj2RcdFlg"
  Relational Operator4/1 -> Switch2/2
  Relational Operator6/1 -> Switch2/1
  Relational Operator5/1 -> Switch3/2
  Relational Operator7/1 -> Switch3/1
  Switch3/1 -> Switch2/3
  Constant4/1 -> Switch3/3
  Constant3/1 -> Switch1/3
  Switch1/1 -> Switch/3
  Switch4/1 -> LM_OTLCurEgoLaObj1RcdFlg/1  "LM_OTLCurEgoLaObj1RcdFlg"
  Relational Operator2/1 -> Switch1/1
  Relational Operator3/1 -> Switch1/2
  Constant2/1 -> Relational Operator3/2
  Subtract1/1 -> Relational Operator2/1
  Relational Operator1/1 -> Switch/1
  Constant1/1 -> Relational Operator1/2, Relational Operator6/2, Relational Operator2/2, Relational Operator7/2
  Subtract/1 -> Relational Operator1/1
  LM_OTLBufEgo2ObjDxK1/1 -> Subtract1/2, Subtract3/2
  LM_OTLCurEgoLaObj1Dx/1 -> Subtract/1, Subtract1/1
  LM_OTLCurEgoLaObj1Index/1 -> Compare To Zero/1
  LM_OTLBufEgo1ObjDxK1/1 -> Subtract/2, Subtract2/2
  Relational Operator/1 -> Switch/2
  Constant/1 -> Relational Operator/2
  LM_OTLCurEgoLaObj1RcdedFlg/1 -> Relational Operator/1, Relational Operator3/1

== system PubIfDecisionLM_MDL/Subsystem2/LM_OTL/LM_OTL_MovObjTrajRecord3/LM_OTL_ObjRcdFlgJudge/LM_OTL_LeLaObjRcdFlgJudge ==
  note: P_LM_OTLTrajPntBaseDis
  LM_OTLCurLeLaObj1RcdedFlg : Inport
  LM_OTLCurLeLaObj2RcdedFlg : Inport  Port=2
  LM_OTLCurLeLaObj1Index : Inport  Port=3
  LM_OTLCurLeLaObj2Index : Inport  Port=4
  LM_OTLCurLeLaObj1Dx : Inport  Port=5
  LM_OTLCurLeLaObj2Dx : Inport  Port=6
  LM_OTLBufLe1ObjDxK1 : Inport  Port=7
  LM_OTLBufLe2ObjDxK1 : Inport  Port=8
  Compare To Zero : simulink/Logic and Bit Operations/Compare To Zero  relop===  OutDataTypeStr=boolean
  Compare To Zero1 : simulink/Logic and Bit Operations/Compare To Zero  relop===  OutDataTypeStr=boolean
  Constant : Constant  OutDataTypeStr=uint8
  Constant1 : Constant  Value=P_LM_OTLTrajPntBaseDis
  Constant2 : Constant  Value=2  OutDataTypeStr=uint8
  Constant3 : Constant  OutDataTypeStr=boolean
  Constant4 : Constant  OutDataTypeStr=boolean
  Constant5 : Constant  OutDataTypeStr=uint8
  Constant6 : Constant  Value=2  OutDataTypeStr=uint8
  Constant7 : Constant  Value=0  OutDataTypeStr=boolean
  DocBlock : simulink/Model-Wide Utilities/DocBlock  DocumentType=Text
      content=|
      | 1.功能描述
      |
      |    该模块的主要功能是判断感兴趣目标当前周期是否满足存储条件
      |
      | 2.算法说明
      |
      |    1）当目标索引不为0
      |    1.1）当目标已经在buffer中存储，需要判断当前dx与上一记录dx的差值是否大于等于2m，满足则置存储标志位为1，否则置0
      |    1.2）当目标未在buffer中存储，则直接置存储标志位为1
      |    2）当目标索引为0（即对应车道不存在感兴趣目标）
      |    直接置存储标志位为0
  Relational Operator{,3..5} (4 alike) : RelationalOperator  Operator===  OutDataTypeStr=boolean  RndMeth=Simplest
  Relational Operator{1..2,6..7} (4 alike) : RelationalOperator  OutDataTypeStr=boolean  RndMeth=Simplest
  Subtract{,1..3} (4 alike) : Sum  Inputs=+-
  Switch{,1..4,7} (6 alike) : Switch  Criteria=u2 ~= 0
  LM_OTLCurLeLaObj1RcdFlg : Outport
  LM_OTLCurLeLaObj2RcdFlg : Outport  Port=2
  wires:
  LM_OTLCurLeLaObj1RcdedFlg/1 -> Relational Operator3/1, Relational Operator/1
  Constant/1 -> Relational Operator/2
  Relational Operator/1 -> Switch/2
  LM_OTLBufLe1ObjDxK1/1 -> Subtract2/2, Subtract/2
  LM_OTLCurLeLaObj1Index/1 -> Compare To Zero/1
  LM_OTLCurLeLaObj1Dx/1 -> Subtract1/1, Subtract/1
  LM_OTLBufLe2ObjDxK1/1 -> Subtract3/2, Subtract1/2
  Subtract/1 -> Relational Operator1/1
  Constant1/1 -> Relational Operator7/2, Relational Operator2/2, Relational Operator6/2, Relational Operator1/2
  Relational Operator1/1 -> Switch/1
  Subtract1/1 -> Relational Operator2/1
  Constant2/1 -> Relational Operator3/2
  Relational Operator3/1 -> Switch1/2
  Relational Operator2/1 -> Switch1/1
  Switch4/1 -> LM_OTLCurLeLaObj1RcdFlg/1  "LM_OTLCurLeLaObj1RcdFlg"
  Switch1/1 -> Switch/3
  Constant3/1 -> Switch1/3
  Constant4/1 -> Switch3/3
  Switch3/1 -> Switch2/3
  Relational Operator7/1 -> Switch3/1
  Relational Operator5/1 -> Switch3/2
  Relational Operator6/1 -> Switch2/1
  Relational Operator4/1 -> Switch2/2
  Switch7/1 -> LM_OTLCurLeLaObj2RcdFlg/1  "LM_OTLCurLeLaObj2RcdFlg"
  Constant6/1 -> Relational Operator5/2
  Constant5/1 -> Relational Operator4/2
  LM_OTLCurLeLaObj2RcdedFlg/1 -> Relational Operator4/1, Relational Operator5/1
  LM_OTLCurLeLaObj2Index/1 -> Compare To Zero1/1
  LM_OTLCurLeLaObj2Dx/1 -> Subtract3/1, Subtract2/1
  Subtract2/1 -> Relational Operator6/1
  Subtract3/1 -> Relational Operator7/1
  Compare To Zero/1 -> Switch4/2
  Constant7/1 -> Switch7/1, Switch4/1
  Switch/1 -> Switch4/3  "LM_OTLLe1ObjRcdValid"
  Compare To Zero1/1 -> Switch7/2
  Switch2/1 -> Switch7/3  "LM_OTLLe1ObjRcdValid"

== system PubIfDecisionLM_MDL/Subsystem2/LM_OTL/LM_OTL_MovObjTrajRecord3/LM_OTL_ObjRcdFlgJudge/LM_OTL_RigLaObjRcdFlgJudge ==
  note: P_LM_OTLTrajPntBaseDis
  LM_OTLCurRigLaObj1Index : Inport
  LM_OTLCurRigLaObj2Index : Inport  Port=2
  LM_OTLCurRigLaObj1Dx : Inport  Port=3
  LM_OTLCurRigLaObj2Dx : Inport  Port=4
  LM_OTLBufRig1ObjDxK1 : Inport  Port=5
  LM_OTLBufRig2ObjDxK1 : Inport  Port=6
  LM_OTLCurRigLaObj1RcdedFlg : Inport  Port=7
  LM_OTLCurRigLaObj2RcdedFlg : Inport  Port=8
  Compare To Zero : simulink/Logic and Bit Operations/Compare To Zero  relop===  OutDataTypeStr=boolean
  Compare To Zero1 : simulink/Logic and Bit Operations/Compare To Zero  relop===  OutDataTypeStr=boolean
  Constant : Constant  OutDataTypeStr=uint8
  Constant1 : Constant  Value=P_LM_OTLTrajPntBaseDis
  Constant2 : Constant  Value=2  OutDataTypeStr=uint8
  Constant3 : Constant  OutDataTypeStr=boolean
  Constant4 : Constant  OutDataTypeStr=boolean
  Constant5 : Constant  OutDataTypeStr=uint8
  Constant6 : Constant  Value=2  OutDataTypeStr=uint8
  Constant7 : Constant  Value=0  OutDataTypeStr=boolean
  DocBlock : simulink/Model-Wide Utilities/DocBlock  DocumentType=Text
      content=|
      | 1.功能描述
      |
      |    该模块的主要功能是判断感兴趣目标当前周期是否满足存储条件
      |
      | 2.算法说明
      |
      |    1）当目标索引不为0
      |    1.1）当目标已经在buffer中存储，需要判断当前dx与上一记录dx的差值是否大于等于2m，满足则置存储标志位为1，否则置0
      |    1.2）当目标未在buffer中存储，则直接置存储标志位为1
      |    2）当目标索引为0（即对应车道不存在感兴趣目标）
      |    直接置存储标志位为0
  Relational Operator{,3..5} (4 alike) : RelationalOperator  Operator===  OutDataTypeStr=boolean  RndMeth=Simplest
  Relational Operator{1..2,6..7} (4 alike) : RelationalOperator  OutDataTypeStr=boolean  RndMeth=Simplest
  Subtract{,1..3} (4 alike) : Sum  Inputs=+-
  Switch{,1..4,7} (6 alike) : Switch  Criteria=u2 ~= 0
  LM_OTLCurRigLaObj1RcdFlg : Outport
  LM_OTLCurRigLaObj2RcdFlg : Outport  Port=2
  wires:
  LM_OTLCurRigLaObj1RcdedFlg/1 -> Relational Operator3/1, Relational Operator/1
  Constant/1 -> Relational Operator/2
  Relational Operator/1 -> Switch/2
  LM_OTLBufRig1ObjDxK1/1 -> Subtract2/2, Subtract/2
  LM_OTLCurRigLaObj1Index/1 -> Compare To Zero/1
  LM_OTLCurRigLaObj1Dx/1 -> Subtract1/1, Subtract/1
  LM_OTLBufRig2ObjDxK1/1 -> Subtract3/2, Subtract1/2
  Subtract/1 -> Relational Operator1/1
  Constant1/1 -> Relational Operator7/2, Relational Operator2/2, Relational Operator6/2, Relational Operator1/2
  Relational Operator1/1 -> Switch/1
  Subtract1/1 -> Relational Operator2/1
  Constant2/1 -> Relational Operator3/2
  Relational Operator3/1 -> Switch1/2
  Relational Operator2/1 -> Switch1/1
  Switch4/1 -> LM_OTLCurRigLaObj1RcdFlg/1  "LM_OTLCurRigLaObj1RcdFlg"
  Switch1/1 -> Switch/3
  Constant3/1 -> Switch1/3
  Constant4/1 -> Switch3/3
  Switch3/1 -> Switch2/3
  Relational Operator7/1 -> Switch3/1
  Relational Operator5/1 -> Switch3/2
  Relational Operator6/1 -> Switch2/1
  Relational Operator4/1 -> Switch2/2
  Switch7/1 -> LM_OTLCurRigLaObj2RcdFlg/1  "LM_OTLCurRigLaObj2RcdFlg"
  Constant6/1 -> Relational Operator5/2
  Constant5/1 -> Relational Operator4/2
  LM_OTLCurRigLaObj2RcdedFlg/1 -> Relational Operator4/1, Relational Operator5/1
  LM_OTLCurRigLaObj2Index/1 -> Compare To Zero1/1
  LM_OTLCurRigLaObj2Dx/1 -> Subtract3/1, Subtract2/1
  Subtract2/1 -> Relational Operator6/1
  Subtract3/1 -> Relational Operator7/1
  Compare To Zero/1 -> Switch4/2
  Constant7/1 -> Switch7/1, Switch4/1
  Switch/1 -> Switch4/3  "LM_OTLEgo1ObjRcdValid"
  Compare To Zero1/1 -> Switch7/2
  Switch2/1 -> Switch7/3  "LM_OTLEgo2ObjRcdValid"

== system PubIfDecisionLM_MDL/Subsystem2/LM_OTL/LM_OTL_MovObjTrajRecord3/LM_OTL_ObjStoreInfoCalc/LM_OTL_BufLe1InfoUpdate1 ==
  LM_OTLBufIndex : Inport
  LM_OTLBufL1DxVectK1Adju : Inport  Port=2
  LM_OTLBufL1DyVectK1Adju : Inport  Port=3
  LM_OTLCurLeLaObj1RcdedFlg : Inport  Port=4
  LM_OTLCurLeLaObj2RcdedFlg : Inport  Port=5
  LM_OTLCurLeLaObj1RcdFlg : Inport  Port=6
  LM_OTLCurLeLaObj2RcdFlg : Inport  Port=7
  LM_OTLCurLeLaObj1ID : Inport  Port=8
  LM_OTLCurLeLaObj2ID : Inport  Port=9
  LM_OTLCurLeLaObj1Dx : Inport  Port=10
  LM_OTLCurLeLaObj2Dx : Inport  Port=11
  LM_OTLCurLeLaObj1Dy : Inport  Port=12
  LM_OTLCurLeLaObj2Dy : Inport  Port=13
  LM_OTLBufL1PNumK1 : Inport  Port=14
  LM_OTLBufL1SPPosK1 : Inport  Port=15
  LM_OTLBufL1EPPosK1 : Inport  Port=16
  LM_OTLCurLeLaObj1Index : Inport  Port=17
  LM_OTLCurLeLaObj2Index : Inport  Port=18
  LM_OTLBufL1LastTPValid : Inport  Port=19
  LM_OTLBufL1LastEPPos : Inport  Port=20
  LM_OTL_BufLe1InfoUpdate : Subsystem
  LM_OTL_BufLe1StoreInfoCalc : Subsystem
  LM_OTLBufL1DxVect : Outport
  LM_OTLBufL1DyVect : Outport  Port=2
  LM_OTLBufL1ObjID : Outport  Port=3
  LM_OTLBufL1EPPos : Outport  Port=4
  LM_OTLBufL1ObjTPNum : Outport  Port=5
  LM_OTLBufL1SPPos : Outport  Port=6
  wires:
  LM_OTLBufIndex/1 -> LM_OTL_BufLe1StoreInfoCalc/1(LM_OTLBufIndex)
  LM_OTLBufL1DxVectK1Adju/1 -> LM_OTL_BufLe1InfoUpdate/1(LM_OTLBufL1DxVectK1Adju)
  LM_OTLCurLeLaObj1Dx/1 -> LM_OTL_BufLe1StoreInfoCalc/8(LM_OTLCurLeLaObj1Dx)
  LM_OTL_BufLe1StoreInfoCalc/5(LM_OTLBufL1ObjID) -> LM_OTLBufL1ObjID/1
  LM_OTL_BufLe1StoreInfoCalc/2(LM_OTLBufL1Objdx) -> LM_OTL_BufLe1InfoUpdate/4(LM_OTLBufL1Objdx)
  LM_OTL_BufLe1StoreInfoCalc/7(LM_OTLBufL1SPPos) -> LM_OTLBufL1SPPos/1
  LM_OTLBufL1EPPosK1/1 -> LM_OTL_BufLe1StoreInfoCalc/14(LM_OTLBufL1EPPosK1)
  LM_OTL_BufLe1InfoUpdate/1(LM_OTLBufL1DxVect) -> LM_OTLBufL1DxVect/1
  LM_OTLCurLeLaObj1RcdedFlg/1 -> LM_OTL_BufLe1StoreInfoCalc/2(LM_OTLCurLeLaObj1RcdedFlg)
  LM_OTLCurLeLaObj1RcdFlg/1 -> LM_OTL_BufLe1StoreInfoCalc/4(LM_OTLCurLeLaObj1RcdFlg)
  LM_OTL_BufLe1InfoUpdate/2(LM_OTLBufL1DyVect) -> LM_OTLBufL1DyVect/1
  LM_OTLCurLeLaObj1Dy/1 -> LM_OTL_BufLe1StoreInfoCalc/10(LM_OTLCurLeLaObj1Dy)
  LM_OTLCurLeLaObj2ID/1 -> LM_OTL_BufLe1StoreInfoCalc/7(LM_OTLCurLeLaObj2ID)
  LM_OTL_BufLe1StoreInfoCalc/4(LM_OTLBufL1EPPos) -> LM_OTL_BufLe1InfoUpdate/6(LM_OTLBufL1EPPos), LM_OTLBufL1EPPos/1
  LM_OTL_BufLe1StoreInfoCalc/6(LM_OTLBufL1ObjTPNum) -> LM_OTLBufL1ObjTPNum/1
  LM_OTLBufL1SPPosK1/1 -> LM_OTL_BufLe1StoreInfoCalc/13(LM_OTLBufL1SPPosK1)
  LM_OTLBufL1DyVectK1Adju/1 -> LM_OTL_BufLe1InfoUpdate/2(LM_OTLBufL1DyVectK1Adju)
  LM_OTL_BufLe1StoreInfoCalc/3(LM_OTLBufL1Objdy) -> LM_OTL_BufLe1InfoUpdate/5(LM_OTLBufL1Objdy)
  LM_OTL_BufLe1StoreInfoCalc/1(LM_OTLBufL1UpdateFlg) -> LM_OTL_BufLe1InfoUpdate/3(LM_OTLBufL1UpdateFlg)
  LM_OTLCurLeLaObj1ID/1 -> LM_OTL_BufLe1StoreInfoCalc/6(LM_OTLCurLeLaObj1ID)
  LM_OTLCurLeLaObj2Dy/1 -> LM_OTL_BufLe1StoreInfoCalc/11(LM_OTLCurLeLaObj2Dy)
  LM_OTLBufL1PNumK1/1 -> LM_OTL_BufLe1StoreInfoCalc/12(LM_OTLBufL1PNumK1)
  LM_OTLCurLeLaObj2Index/1 -> LM_OTL_BufLe1StoreInfoCalc/16(LM_OTLCurLeLaObj2Index)
  LM_OTLCurLeLaObj1Index/1 -> LM_OTL_BufLe1StoreInfoCalc/15(LM_OTLCurLeLaObj1Index)
  LM_OTLCurLeLaObj2RcdedFlg/1 -> LM_OTL_BufLe1StoreInfoCalc/3(LM_OTLCurLeLaObj2RcdedFlg)
  LM_OTLBufL1LastTPValid/1 -> LM_OTL_BufLe1StoreInfoCalc/17(LM_OTLBufL1LastTPValid)
  LM_OTLBufL1LastEPPos/1 -> LM_OTL_BufLe1StoreInfoCalc/18(LM_OTLBufL1LastEPPos)
  LM_OTLCurLeLaObj2RcdFlg/1 -> LM_OTL_BufLe1StoreInfoCalc/5(LM_OTLCurLeLaObj2RcdFlg)
  LM_OTLCurLeLaObj2Dx/1 -> LM_OTL_BufLe1StoreInfoCalc/9(LM_OTLCurLeLaObj2Dx)

== system PubIfDecisionLM_MDL/Subsystem2/LM_OTL/LM_OTL_MovObjTrajRecord3/LM_OTL_ObjStoreInfoCalc/Subsystem ==
  LM_OTLBufL1DxVect : Inport
  LM_OTLBufL1DyVect : Inport  Port=2
  LM_OTLBufL1ObjID : Inport  Port=3
  LM_OTLBufL1EPPos : Inport  Port=4
  LM_OTLBufL1ObjTPNum : Inport  Port=5
  LM_OTLBufL1SPPos : Inport  Port=6
  LM_OTLBufL2DxVect : Inport  Port=7
  LM_OTLBufL2DyVect : Inport  Port=8
  LM_OTLBufL2ObjID : Inport  Port=9
  LM_OTLBufL2EPPos : Inport  Port=10
  LM_OTLBufL2ObjTPNum : Inport  Port=11
  LM_OTLBufL2SPPos : Inport  Port=12
  LM_OTLBufE1DxVect : Inport  Port=13
  LM_OTLBufE1DyVect : Inport  Port=14
  LM_OTLBufE1ObjID : Inport  Port=15
  LM_OTLBufE1EPPos : Inport  Port=16
  LM_OTLBufE1ObjTPNum : Inport  Port=17
  LM_OTLBufE1SPPos : Inport  Port=18
  LM_OTLBufE2DxVect : Inport  Port=19
  LM_OTLBufE2DyVect : Inport  Port=20
  LM_OTLBufE2ObjID : Inport  Port=21
  LM_OTLBufE2EPPos : Inport  Port=22
  LM_OTLBufE2ObjTPNum : Inport  Port=23
  LM_OTLBufLE2SPPos : Inport  Port=24
  LM_OTLBufR1DxVect : Inport  Port=25
  LM_OTLBufR1DyVect : Inport  Port=26
  LM_OTLBufR1ObjID : Inport  Port=27
  LM_OTLBufR1EPPos : Inport  Port=28
  LM_OTLBufR1ObjTPNum : Inport  Port=29
  LM_OTLBufR1SPPos : Inport  Port=30
  LM_OTLBufR2DxVect : Inport  Port=31
  LM_OTLBufR2DyVect : Inport  Port=32
  LM_OTLBufR2ObjID : Inport  Port=33
  LM_OTLBufR2EPPos : Inport  Port=34
  LM_OTLBufR2ObjTPNum : Inport  Port=35
  LM_OTLBufR2SPPos : Inport  Port=36
  LM_OTLBufLastTPInfoBus : Inport  Port=37
  LM_OTL_BufEPPosInfo : Subsystem
  LM_OTL_BufLastTPInfo : Subsystem
  LM_OTL_BufObjIDInfo : Subsystem
  LM_OTL_BufPNumInfo : Subsystem
  LM_OTL_BufSPPosInfo : Subsystem
  LM_OTL_BufTPVectInfo : Subsystem
  Subsystem1 : Subsystem
  LM_OTLBufTPVectBus : Outport
  LM_OTLBufTPInfoBus : Outport  Port=2
  wires:
  LM_OTLBufL1DxVect/1 -> [LM_OTLBufL1DxVect], LM_OTL_BufTPVectInfo/1(LM_OTLBufL1DxVect)
  LM_OTLBufL1DyVect/1 -> LM_OTL_BufTPVectInfo/2(LM_OTLBufL1DyVect)
  LM_OTLBufL2DxVect/1 -> [LM_OTLBufL2DxVect], LM_OTL_BufTPVectInfo/3(LM_OTLBufL2DxVect)
  LM_OTLBufL2DyVect/1 -> LM_OTL_BufTPVectInfo/4(LM_OTLBufL2DyVect)
  LM_OTLBufE1DxVect/1 -> [LM_OTLBufE1DxVect], LM_OTL_BufTPVectInfo/5(LM_OTLBufE1DxVect)
  LM_OTLBufE1DyVect/1 -> LM_OTL_BufTPVectInfo/6(LM_OTLBufE1DyVect)
  LM_OTLBufE2DxVect/1 -> [LM_OTLBufE2DxVect], LM_OTL_BufTPVectInfo/7(LM_OTLBufE2DxVect)
  LM_OTLBufE2DyVect/1 -> LM_OTL_BufTPVectInfo/8(LM_OTLBufE2DyVect)
  LM_OTLBufR1DxVect/1 -> [LM_OTLBufR1DxVect], LM_OTL_BufTPVectInfo/9(LM_OTLBufR1DxVect)
  LM_OTLBufR1DyVect/1 -> LM_OTL_BufTPVectInfo/10(LM_OTLBufR1DyVect)
  LM_OTLBufR2DxVect/1 -> [LM_OTLBufR2DxVect], LM_OTL_BufTPVectInfo/11(LM_OTLBufR2DxVect)
  LM_OTLBufR2DyVect/1 -> LM_OTL_BufTPVectInfo/12(LM_OTLBufR2DyVect)
  LM_OTL_BufTPVectInfo/1(LM_OTLBufTPVectBus) -> LM_OTL_BufLastTPInfo/2(LM_OTLBufTPVectBus), LM_OTLBufTPVectBus/1
  LM_OTLBufL1ObjID/1 -> LM_OTL_BufObjIDInfo/1(LM_OTLBufL1ObjID)
  LM_OTLBufL2ObjID/1 -> LM_OTL_BufObjIDInfo/2(LM_OTLBufL2ObjID)
  LM_OTLBufE1ObjID/1 -> LM_OTL_BufObjIDInfo/3(LM_OTLBufE1ObjID)
  LM_OTLBufE2ObjID/1 -> LM_OTL_BufObjIDInfo/4(LM_OTLBufE2ObjID)
  LM_OTLBufR1ObjID/1 -> LM_OTL_BufObjIDInfo/5(LM_OTLBufR1ObjID)
  LM_OTLBufR2ObjID/1 -> LM_OTL_BufObjIDInfo/6(LM_OTLBufR2ObjID)
  LM_OTLBufL1ObjTPNum/1 -> LM_OTL_BufPNumInfo/1(LM_OTLBufL1ObjTPNum)
  LM_OTLBufL2ObjTPNum/1 -> LM_OTL_BufPNumInfo/2(LM_OTLBufL2ObjTPNum)
  LM_OTLBufE1ObjTPNum/1 -> LM_OTL_BufPNumInfo/3(LM_OTLBufE1ObjTPNum)
  LM_OTLBufE2ObjTPNum/1 -> LM_OTL_BufPNumInfo/4(LM_OTLBufE2ObjTPNum)
  LM_OTLBufR1ObjTPNum/1 -> LM_OTL_BufPNumInfo/5(LM_OTLBufR1ObjTPNum)
  LM_OTLBufR2ObjTPNum/1 -> LM_OTL_BufPNumInfo/6(LM_OTLBufR2ObjTPNum)
  LM_OTLBufL2SPPos/1 -> LM_OTL_BufSPPosInfo/2(LM_OTLBufL2SPPos)
  LM_OTLBufL1SPPos/1 -> LM_OTL_BufSPPosInfo/1(LM_OTLBufL1SPPos)
  LM_OTLBufE1SPPos/1 -> LM_OTL_BufSPPosInfo/3(LM_OTLBufE1SPPos)
  LM_OTLBufLE2SPPos/1 -> LM_OTL_BufSPPosInfo/4(LM_OTLBufLE2SPPos)
  LM_OTLBufR1SPPos/1 -> LM_OTL_BufSPPosInfo/5(LM_OTLBufR1SPPos)
  LM_OTLBufR2SPPos/1 -> LM_OTL_BufSPPosInfo/6(LM_OTLBufR2SPPos)
  LM_OTLBufL1EPPos/1 -> LM_OTL_BufEPPosInfo/1(LM_OTLBufL1EPPos)
  LM_OTLBufL2EPPos/1 -> LM_OTL_BufEPPosInfo/2(LM_OTLBufL2EPPos)
  LM_OTLBufE2EPPos/1 -> LM_OTL_BufEPPosInfo/4(LM_OTLBufE2EPPos)
  LM_OTLBufR1EPPos/1 -> LM_OTL_BufEPPosInfo/5(LM_OTLBufR1EPPos)
  LM_OTLBufR2EPPos/1 -> LM_OTL_BufEPPosInfo/6(LM_OTLBufR2EPPos)
  LM_OTLBufE1EPPos/1 -> LM_OTL_BufEPPosInfo/3(LM_OTLBufE1EPPos)
  LM_OTLBufLastTPInfoBus/1 -> LM_OTL_BufLastTPInfo/4(LM_OTLBufLastTPInfoBus)
  LM_OTL_BufObjIDInfo/1(LM_OTLBufObjIDInfo) -> Subsystem1/1(LM_OTLBufObjIDInfo)
  LM_OTL_BufPNumInfo/1(LM_OTLBufPNumInfo) -> Subsystem1/2(LM_OTLBufPNumInfo), LM_OTL_BufLastTPInfo/3(LM_OTLBufPNumInfo)
  LM_OTL_BufSPPosInfo/1(LM_OTLBufSPPosInfo) -> Subsystem1/3(LM_OTLBufSPPosInfo)
  LM_OTL_BufEPPosInfo/1(LM_OTLBufEPPosInfo) -> Subsystem1/4(LM_OTLBufEPPosInfo), LM_OTL_BufLastTPInfo/1(LM_OTLBufEPPosInfo)
  LM_OTL_BufLastTPInfo/4(LM_OTLBufLastEPPosInfo) -> Subsystem1/8(LM_OTLBufLastEPPosInfo)
  LM_OTL_BufLastTPInfo/3(LM_OTLBufLastSPPosInfo) -> Subsystem1/7(LM_OTLBufLastSPPosInfo)
  LM_OTL_BufLastTPInfo/2(LM_OTLBufLastPNumInfo) -> Subsystem1/6(LM_OTLBufLastPNumInfo)
  LM_OTL_BufLastTPInfo/1(LM_OTLBufLastTPValid) -> Subsystem1/5(LM_OTLBufLastTPValid)
  Subsystem1/1(LM_OTLBufTPInfoBus) -> LM_OTLBufTPInfoBus/1

== system PubIfDecisionLM_MDL/Subsystem2/LM_SigPrePro1/Subsystem1/Subsystem/Subsystem ==
  RFM_LINE : Inport
  Bus Creator : BusCreator  Inputs=13
  Bus Selector : BusSelector  OutputSignals=dC0V
  Bus Selector1 : BusSelector  OutputSignals=bIsLineExist,dC1V,dC2V,dC3V,dLaneWidth,eLineType,dDisStart,dDisFront,dQuality,eColour,eFuType,nTrackAge
  Constant : Constant  Value=P_LM_VSLMinLINEL1  OutDataTypeStr=single
  Constant1 : Constant  Value=P_LM_VSLMaxLINEL1  OutDataTypeStr=single
  Constant8 : Constant  Value=0  OutDataTypeStr=single
  Logical Operator : Logic  AllPortsSameDT=off  OutDataTypeStr=boolean
  Relational Operator : RelationalOperator  OutDataTypeStr=boolean  RndMeth=Simplest
  Relational Operator1 : RelationalOperator  Operator=<=  OutDataTypeStr=boolean  RndMeth=Simplest
  Switch : Switch  Criteria=u2 > Threshold
  RFM_LINE_L1 : Outport
  wires:
  Relational Operator1/1 -> Logical Operator/2
  Bus Selector1/6 -> Bus Creator/7  "<eLineType>"
  Bus Selector1/8 -> Bus Creator/9  "<dDisFront>"
  Bus Selector1/5 -> Bus Creator/6  "<dLaneWidth>"
  Bus Selector1/9 -> Bus Creator/10  "<dQuality>"
  RFM_LINE/1 -> Bus Selector/1, Bus Selector1/1
  Logical Operator/1 -> Switch/2
  Bus Selector1/1 -> Bus Creator/1  "<bIsLineExist>"
  Bus Selector1/10 -> Bus Creator/11  "<eColour>"
  Bus Selector1/7 -> Bus Creator/8  "<dDisStart>"
  Bus Selector/1 -> Relational Operator1/1, Relational Operator/1, Switch/1  "<dC0V>"
  Switch/1 -> [dC0V]  "dC0V"
  Bus Selector1/3 -> Bus Creator/4  "<dC2V>"
  Bus Selector1/4 -> Bus Creator/5  "<dC3V>"
  Constant1/1 -> Relational Operator1/2
  Relational Operator/1 -> Logical Operator/1
  Constant8/1 -> Switch/3
  Bus Selector1/2 -> Bus Creator/3  "<dC1V>"
  [dC0V] -> Bus Creator/2  "dC0V"
  Constant/1 -> Relational Operator/2
  Bus Creator/1 -> RFM_LINE_L1/1
  Bus Selector1/11 -> Bus Creator/12  "<eFuType>"
  Bus Selector1/12 -> Bus Creator/13  "<nTrackAge>"

== system PubIfDecisionLM_MDL/Subsystem2/LM_SigPrePro1/Subsystem1/Subsystem/Subsystem1 ==
  RFM_LINE : Inport
  Bus Creator : BusCreator  Inputs=13
  Bus Selector : BusSelector  OutputSignals=dC0V
  Bus Selector1 : BusSelector  OutputSignals=bIsLineExist,dC1V,dC2V,dC3V,dLaneWidth,eLineType,dDisStart,dDisFront,dQuality,eColour,eFuType,nTrackAge
  Constant2 : Constant  Value=P_LM_VSLMinLINER1  OutDataTypeStr=single
  Constant3 : Constant  Value=P_LM_VSLMaxLINER1  OutDataTypeStr=single
  Constant8 : Constant  Value=0  OutDataTypeStr=single
  Logical Operator : Logic  AllPortsSameDT=off  OutDataTypeStr=boolean
  Relational Operator : RelationalOperator  OutDataTypeStr=boolean  RndMeth=Simplest
  Relational Operator1 : RelationalOperator  Operator=<=  OutDataTypeStr=boolean  RndMeth=Simplest
  Switch : Switch  Criteria=u2 > Threshold
  RFM_LINE_R1 : Outport
  wires:
  Bus Creator/1 -> RFM_LINE_R1/1
  Constant2/1 -> Relational Operator/2
  [dC0V] -> Bus Creator/2  "dC0V"
  Bus Selector1/2 -> Bus Creator/3  "<dC1V>"
  Constant8/1 -> Switch/3
  Relational Operator/1 -> Logical Operator/1
  Constant3/1 -> Relational Operator1/2
  Bus Selector1/4 -> Bus Creator/5  "<dC3V>"
  Bus Selector1/3 -> Bus Creator/4  "<dC2V>"
  Switch/1 -> [dC0V]  "dC0V"
  Bus Selector/1 -> Switch/1, Relational Operator/1, Relational Operator1/1  "<dC0V>"
  Bus Selector1/7 -> Bus Creator/8  "<dDisStart>"
  Bus Selector1/10 -> Bus Creator/11  "<eColour>"
  Bus Selector1/1 -> Bus Creator/1  "<bIsLineExist>"
  Logical Operator/1 -> Switch/2
  RFM_LINE/1 -> Bus Selector1/1, Bus Selector/1
  Bus Selector1/9 -> Bus Creator/10  "<dQuality>"
  Bus Selector1/5 -> Bus Creator/6  "<dLaneWidth>"
  Bus Selector1/8 -> Bus Creator/9  "<dDisFront>"
  Bus Selector1/6 -> Bus Creator/7  "<eLineType>"
  Relational Operator1/1 -> Logical Operator/2
  Bus Selector1/11 -> Bus Creator/12  "<eFuType>"
  Bus Selector1/12 -> Bus Creator/13  "<nTrackAge>"
